simulink model "model_4"  (R2021b)
settings: Solver=FixedStepAuto  StartTime=0.0  StopTime=20  FixedStep=0.0005  RelTol=1e-3
libraries: cstblocks x1
settings Model: Creator=den  LastModifiedBy=vital

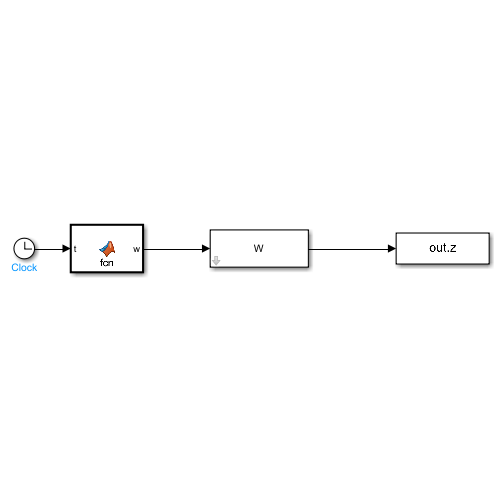
[thumbnail: Simulink's stored preview of the top-level diagram]
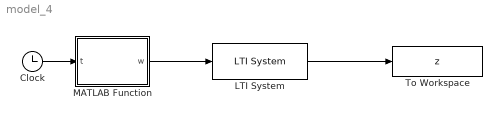
== system model_4 ==
  Clock : Clock
  LTI System : cstblocks/LTI System  sys=W  IC=[]
  MATLAB Function : MATLAB Function  TreatAsAtomicUnit=on
  To Workspace : ToWorkspace  VariableName=z  SaveFormat=Timeseries  SampleTime=-1
  wires:
  LTI System/1 -> To Workspace/1
  MATLAB Function/1(w) -> LTI System/1
  Clock/1 -> MATLAB Function/1(t)

== matlab function model_4/MATLAB Function ==
  data: t input; w output
function w = fcn(t)

w = [sin(6*t); 2*cos(6*t); 3*sin(6*t+pi/4)];
